simulink model "Temporal4_2018a"  (R2018a)
settings: Solver=VariableStepAuto  StartTime=0.0  StopTime=1.0  RelTol=1e-3
settings Model: Creator=86188  LastModifiedBy=bzhan

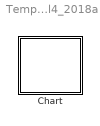
== system Temporal4_2018a ==
  Chart : Stateflow chart  TreatAsAtomicUnit=on

== stateflow chart Temporal4_2018a/Chart ==
  settings: updateMethod=DISCRETE  sampleTime=0.1
  state A
    en:f("en_A");
    x=1;
    du:f("du_A");
    x=x+1;
  state B
    en:f("en_B")
    x=1;
    du:f("du_B");
    x=x+1;
  (default) -> A
  A -> B : before(4,tick)[x>=3]
  B -> A : before(4,tick)[x>=4]
  data: s function_input; x local
  function f(s):
    | function f(s)
    |   fprintf(s+"\n");
